simulink model "FLCU_Gauging_Test_Harness_Converting"  (R2019b)
settings: Solver=FixedStepAuto  StartTime=0.0  StopTime=10  FixedStep=0.02  RelTol=1e-3
settings Model: DataDictionary=FLCU_Gauging.sldd  Creator=aymanouchker  LastModifiedBy=aymanouchker
settings DataIOCC: SignalLoggingName=BusData
settings OptimizationCC: DefaultParameterBehavior=Inlined  UseDivisionForNetSlopeComputation=on  GainParamInheritBuiltInType=on  UseFloatMulNetSlope=on  DefaultUnderspecifiedDataType=single  UseSpecifiedMinMax=on  InlineInvariantSignals=on  EnhancedBackFolding=on  CachingGlobalReferences=on  PassReuseOutputArgsAs=Individual arguments  StateBitsets=on  DataBitsets=on  ZeroExternalMemoryAtStartup=off  ZeroInternalMemoryAtStartup=off  NoFixptDivByZeroProtection=on  EfficientFloat2IntCast=on  LifeSpan=inf  OptimizeBlockOrder=speed  DifferentSizesBufferReuse=on  EfficientTunableParamExpr=on
settings DebuggingCC: SignalInfNanChecking=warning  IntegerOverflowMsg=error  ParameterTunabilityLossMsg=error  UniqueDataStoreMsg=error  AssertControl=DisableAll  StrictBusMsg=ErrorOnBusTreatedAsVector  SFUndirectedBroadcastEventsDiag=error
settings HardwareCC: ProdBitPerInt=16  ProdBitPerPointer=16  ProdBitPerSizeT=16  ProdBitPerPtrDiffT=16  ProdLargestAtomicFloat=None  ProdWordSize=16  ProdLongLongMode=on  ProdHWDeviceType=STMicroelectronics->ST10/Super10
settings SFSimCC: CompileTimeRecursionLimit=0  EnableRuntimeRecursion=off  MATLABDynamicMemAlloc=off
settings RTWCC: SystemTargetFile=ert.tlc  TemplateMakefile=ert_default_tmf  GenerateReport=on  BuildConfiguration=Faster Runs  IncludeHyperlinkInReport=on  LaunchReport=on  GenerateTraceInfo=on  GenerateTraceReport=on  GenerateTraceReportSl=on  GenerateTraceReportSf=on  GenerateTraceReportEml=on
settings CodeAppCC: ForceParamTrailComments=on  IgnoreCustomStorageClasses=off  IgnoreTestpoints=on  OperatorAnnotations=on  SimulinkDataObjDesc=on  SFDataObjDesc=on  MATLABFcnDesc=on  InsertBlockDesc=on  StateflowObjectComments=on  MATLABSourceComments=on  EnableCustomComments=on  ReqsInCode=on
settings ERTTargetCC: TargetLangStandard=C99 (ISO)  UtilityFuncGeneration=Shared location  GenerateSampleERTMain=on  CombineSignalStateStructs=on  SuppressErrorStatus=on  SupportAbsoluteTime=off  MultiInstanceERTCode=on  CodeInterfacePackaging=Reusable function  SupportNonFinite=off  ParenthesesLevel=Maximum  CastingMode=Standards  GenerateSharedConstants=off  InlinedParameterPlacement=NonHierarchical  ERTCustomFileTemplate=example_file_process.tlc  PreserveExpressionOrder=on  PreserveIfCondition=on  EnableSignedLeftShifts=off  EnableSignedRightShifts=off

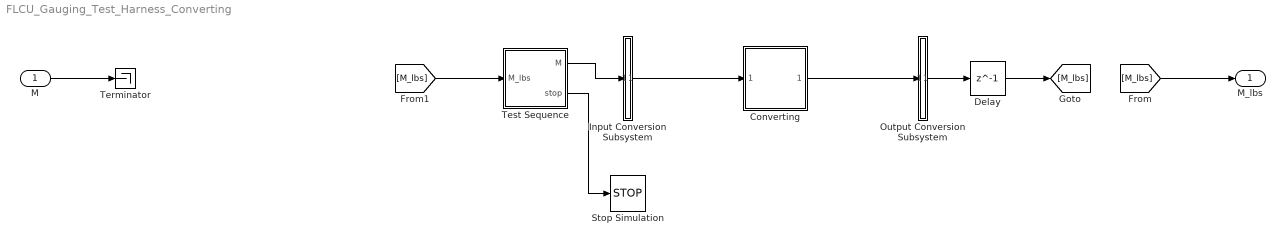
== system FLCU_Gauging_Test_Harness_Converting ==
  M : Inport  OutDataTypeStr=double  PortDimensions=[1]  SampleTime=0.02
  Converting : Subsystem  Tag=__SL_testing_harness_stub_
  Delay : Delay  DelayLength=1
  Input Conversion Subsystem : Subsystem  Tag=__SLT_ICS__  Description=|
      | Signal spec.
      | and routing
      settings: AttributesFormatString=%<Description>
  Output Conversion Subsystem : Subsystem  Tag=__SLT_OCS__  Description=|
      | Signal spec.
      | and routing
      settings: AttributesFormatString=%<Description>
  Stop Simulation : Stop
  Terminator : Terminator
  Test Sequence : Test Sequence  TreatAsAtomicUnit=on
  M_lbs : Outport
  wires:
  Input Conversion Subsystem/1(Outport_1) -> Converting/1(harness_in_1)
  Converting/1(harness_out_1) -> Output Conversion Subsystem/1(Inport_1)
  M/1 -> Terminator/1
  Output Conversion Subsystem/1(Outport_1) -> Delay/1
  Delay/1 -> [M_lbs]
  [M_lbs] -> M_lbs/1
  [M_lbs] -> Test Sequence/1(M_lbs)
  Test Sequence/1(M) -> Input Conversion Subsystem/1(Inport_1)
  Test Sequence/2(stop) -> Stop Simulation/1

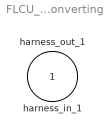
== system FLCU_Gauging_Test_Harness_Converting/Converting ==
  harness_in_1 : Inport
  harness_out_1 : Outport

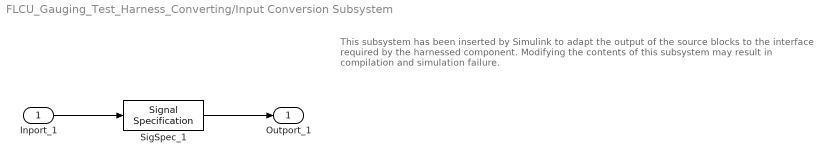
== system FLCU_Gauging_Test_Harness_Converting/Input Conversion Subsystem ==
  note: This subsystem has been inserted by Simulink to adapt the output of the source blocks to the interface required by the harnessed component.
      |  Modifying the contents of this subsystem may result in compilation and simulation failure.
  Inport_1 : Inport
  SigSpec_1 : SignalSpecification  OutDataTypeStr=double  Unit=kg  Dimensions=[1]  SampleTime=0.02
  Outport_1 : Outport
  wires:
  SigSpec_1/1 -> Outport_1/1
  Inport_1/1 -> SigSpec_1/1

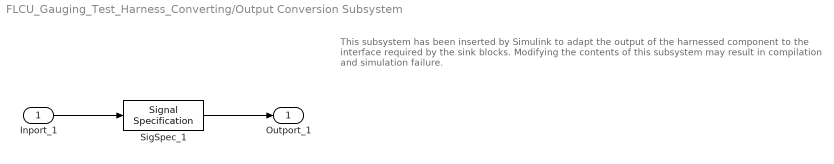
== system FLCU_Gauging_Test_Harness_Converting/Output Conversion Subsystem ==
  note: This subsystem has been inserted by Simulink to adapt the output of the harnessed component to the interface required by the sink blocks.
      |  Modifying the contents of this subsystem may result in compilation and simulation failure.
  Inport_1 : Inport
  SigSpec_1 : SignalSpecification  OutDataTypeStr=double  Unit=lb  Dimensions=[1]  SampleTime=0.02
  Outport_1 : Outport
  wires:
  Inport_1/1 -> SigSpec_1/1
  SigSpec_1/1 -> Outport_1/1

== stateflow chart FLCU_Gauging_Test_Harness_Converting/Test Sequence ==
  settings: stateMachineType=SIMPLIFIED_MACHINE
  state Initialization
    M=0;
    stop=false;
    count=0;
  state step_1
    M=0;
  state step_2
    verify(M_lbs==0);
  state step_3
    M=1;
  state step_4
    verify(M_lbs==2.205);
  state step_5
    M=-1;
  state step_6
    verify(M_lbs==-2.205);
  state step_7
    stop=true;
  (default) -> Initialization
  Initialization -> step_1
  data: M_lbs input; M output; stop output; count local
